simulink model "W09_E_weather"  (R2024b)
settings: Solver=ode4  StartTime=0  StopTime=T_final  FixedStep=h  RelTol=1e-3
values from neighbouring files (symbols this model uses):
  beta_c = pi/2    (= 1.57079632679)    [W09_0_setup.m]
  Delta = 5    [W09_0_setup.m]
  e_min = 0.3    [W09_0_setup.m]
  h = 0.02    [W09_0_setup.m]    (also in W09_1_build_vessel.m = add_line(sys, [a; via; b]); W09_metrics.m = V.h)
  hand_over = 1    [W09_0_setup.m]
  k_neg = cfg.k_neg    [W09_0_setup.m]
  k_pos = cfg.k_pos    [W09_0_setup.m]
  kappa = 0.3    [W09_0_setup.m]
  Kd = 100    [W09_0_setup.m]
  Kd_x = 60    [W09_0_setup.m]
  Ki_u = 200    [W09_0_setup.m]
  Ki_x = 3    [W09_0_setup.m]
  Kp = 300    [W09_0_setup.m]
  Kp_u = 200    [W09_0_setup.m]
  Kp_x = 30    [W09_0_setup.m]
  mp = 25    [W09_0_setup.m]
  N_max = min(2*cfg.y_pont*(cfg.k_pos*cfg.n_max^2 - X_max/2),              2*cfg.y_pont*(X_max/2 + cfg.k_neg*cfg.n_min^2))    [W09_0_setup.m]
  N_open = 2*cfg.y_pont*cfg.k_pos*cfg.n_max^2    [W09_0_setup.m]
  phi_i = mod(phi_i + phase_shift, 2*pi)    [W09_0_setup.m]
  R_arrive = 3    [W09_0_setup.m]
  rp = [0.05 0 -0.35]'    [W09_0_setup.m]
  T_hold = 30    [W09_0_setup.m]
  T_max = cfg.k_pos*cfg.n_max^2    [W09_0_setup.m]
  T_min = -cfg.k_neg*cfg.n_min^2    [W09_0_setup.m]
  u_d = 1.0    (= 1)    [W09_0_setup.m]
  use_ilos = 1    [W09_0_setup.m]
  use_Kd = 1    [W09_0_setup.m]
  use_Ki_u = 1    [W09_0_setup.m]
  use_pass = 1    [W09_0_setup.m]
  use_scale = 1    [W09_0_setup.m]
  use_ssa = 1    [W09_0_setup.m]
  use_vane = 1    [W09_0_setup.m]
  V_c = 0.3    [W09_0_setup.m]
  w0 = 2*pi/T0    (= 3.14159265359)    [W09_0_setup.m]
  wave_on = 1    [W09_0_setup.m]
  WP_E = [ 0 60 60]'    [W09_0_setup.m]
  WP_N = [60 60  0]'    [W09_0_setup.m]
  x0 = zeros(12,1)    [W09_0_setup.m]
  X_max = 120    [W09_0_setup.m]
  y_pont = cfg.y_pont    [W09_0_setup.m]
  zeta_d = 0.3    [W09_0_setup.m]
  zeta_n = 0.05    [W09_0_setup.m]
undefined symbols (not defined in the file or in its folder): a_i, k_w, w_i
settings Model: Creator=admin  LastModifiedBy=admin
settings DataIOCC: ReturnWorkspaceOutputs=off

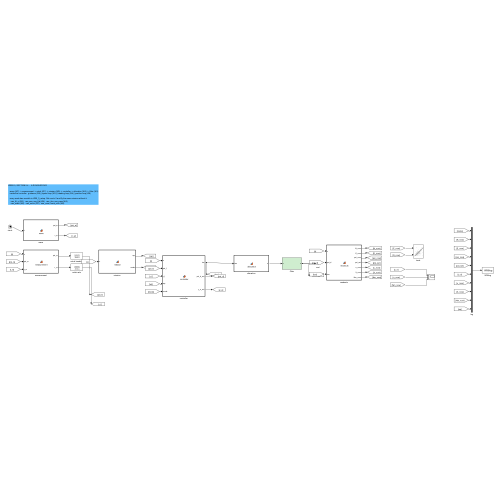
[thumbnail: Simulink's stored preview of the top-level diagram]
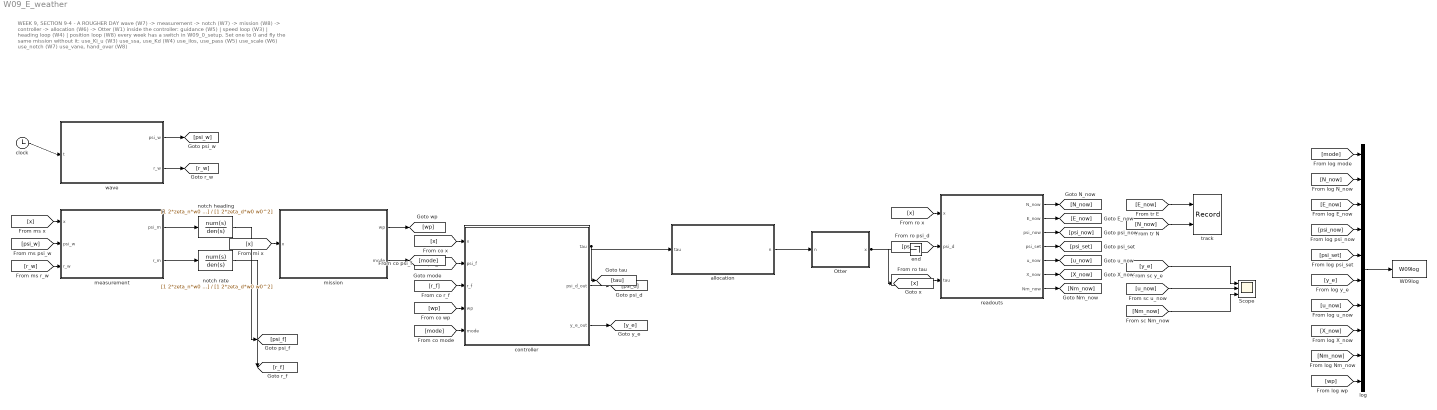
== system W09_E_weather ==
  note: WEEK 9, SECTION 9-4  -  A ROUGHER DAY
      |
      |    wave (W7) -> measurement -> notch (W7) -> mission (W8) -> controller -> allocation (W6) -> Otter (W1)
      |    inside the controller:  guidance (W5) | speed loop (W3) | heading loop (W4) | position loop (W8)
      |
      |    every week has a switch in W09_0_setup. Set one to 0 and fly the same mission without it:
      |      use_Ki_u (W3)   use_ssa, use_Kd (W4)   use_ilos, use_pass (W5)
      |      use_scale (W6)   use_notch (W7)   use_vane, hand_over (W8)
  Otter : Subsystem
  Scope : Scope  NumInputPorts=3
  W09log : ToWorkspace  VariableName=W09log  SaveFormat=Structure With Time  SampleTime=-1
  allocation : MATLAB Function  TreatAsAtomicUnit=on
  clock : Clock
  controller : MATLAB Function  TreatAsAtomicUnit=on
  end : Terminator
  log : Mux  Inputs=10
  measurement : MATLAB Function  TreatAsAtomicUnit=on
  mission : MATLAB Function  TreatAsAtomicUnit=on
  notch heading : TransferFcn  Numerator=[1 2*zeta_n*w0 w0^2]  Denominator=[1 2*zeta_d*w0 w0^2]
  notch rate : TransferFcn  Numerator=[1 2*zeta_n*w0 w0^2]  Denominator=[1 2*zeta_d*w0 w0^2]
  readouts : MATLAB Function  TreatAsAtomicUnit=on
  track : Record  FileSettingsInternal="{\"entries\":[{\"content\":{\"excelSettings\":{\"content\":{},\"type\":\"Streamout.ExcelSettings\"}},\"type\":\"Streamout.FileSettingStorage\",\"uuid\":\"\"}],\"packageUris\":[\"http:\\/\\/schema.mathworks.com\\/mf0\\/streamout_blocks\\/R2020a\"],\"version\":\"1.0\"}"  Layout=[1 1]  SignalsInternal="{\"entries\":[{\"content\":{\"signals\":[{\"content\":{\"blockPath\":[],\"dimensions\":[1],\"domain\":\"\",\"lineColor\":\"#a2142f\",\"plots\":[ 1 ],\"port\":1,\"signalID\":1,\"signalName\":\"XY Graph:1\"},\"type\":\"RecordBlkView.Signal\",\"uuid\":\"\"},{\"content\":{\"blockPath\":[],\"dimensions\":[1],\"domain\":\"\",\"lineColor\":\"#139fff\",\"plots\":[ 1 ],\"port\":2,\"signalID\":2,\"signalName\":\"XY Graph:2\"},\"type\":\"RecordBlkView.Signal\",\"uuid\":\"\"}]},\"type\":\"RecordBlkView.InputSignals\",\"uuid\":\"\"}],\"packageUris\":[\"http:\\/\\/schema.mathworks.com\\/mf0\\/streamout_blocks\\/R2020a\"],\"version\":\"1.0\"}"  VisualizationBindings="{\"xyplotplugin\":{\"info\":[{\"series\":[{\"bindingParametersList\":[{\"parameter\":\"X-Axis\",\"signalID\":1,\"signalName\":\"XY Graph:1\"},{\"parameter\":\"Y-Axis\",\"signalID\":2,\"signalName\":\"XY Graph:2\"}],\"seriesID\":0}],\"subplotID\":1}]}}"  CompatibilityTag=XY
  wave : MATLAB Function  TreatAsAtomicUnit=on
  wires:
  clock/1 -> wave/1(t)
  wave/1(psi_w) -> [psi_w]
  wave/2(r_w) -> [r_w]
  [x] -> measurement/1(x)
  [psi_w] -> measurement/2(psi_w)
  [r_w] -> measurement/3(r_w)
  measurement/1(psi_m) -> notch heading/1
  notch heading/1 -> [psi_f]
  measurement/2(r_m) -> notch rate/1
  notch rate/1 -> [r_f]
  [x] -> mission/1(x)
  mission/1(wp) -> [wp]
  mission/2(mode) -> [mode]
  [x] -> controller/1(x)
  [psi_f] -> controller/2(psi_f)
  [r_f] -> controller/3(r_f)
  [wp] -> controller/4(wp)
  [mode] -> controller/5(mode)
  controller/1(tau) -> [tau], allocation/1(tau)
  controller/2(psi_d_out) -> [psi_d]
  controller/3(y_e_out) -> [y_e]
  allocation/1(n) -> Otter/1(n)
  Otter/1(x) -> [x], end/1
  [x] -> readouts/1(x)
  [psi_d] -> readouts/2(psi_d)
  [tau] -> readouts/3(tau)
  readouts/1(N_now) -> [N_now]
  readouts/2(E_now) -> [E_now]
  readouts/3(psi_now) -> [psi_now]
  readouts/4(psi_set) -> [psi_set]
  readouts/5(u_now) -> [u_now]
  readouts/6(X_now) -> [X_now]
  readouts/7(Nm_now) -> [Nm_now]
  [E_now] -> track/1
  [N_now] -> track/2
  [y_e] -> Scope/1
  [u_now] -> Scope/2
  [Nm_now] -> Scope/3
  [mode] -> log/1
  [N_now] -> log/2
  [E_now] -> log/3
  [psi_now] -> log/4
  [psi_set] -> log/5
  [y_e] -> log/6
  [u_now] -> log/7
  [X_now] -> log/8
  [Nm_now] -> log/9
  [wp] -> log/10
  log/1 -> W09log/1

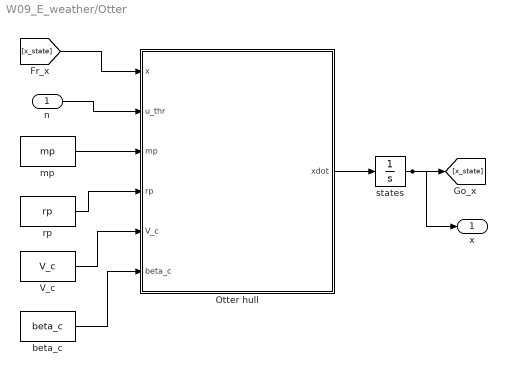
== system W09_E_weather/Otter ==
  n : Inport
  Otter hull : MATLAB Function  TreatAsAtomicUnit=on
  V_c : Constant  Value=V_c
  beta_c : Constant  Value=beta_c
  mp : Constant  Value=mp
  rp : Constant  Value=rp
  states : Integrator  InitialCondition=x0
  x : Outport
  wires:
  states/1 -> [x_state], x/1
  Otter hull/1(xdot) -> states/1
  [x_state] -> Otter hull/1(x)
  n/1 -> Otter hull/2(u_thr)
  mp/1 -> Otter hull/3(mp)
  rp/1 -> Otter hull/4(rp)
  V_c/1 -> Otter hull/5(V_c)
  beta_c/1 -> Otter hull/6(beta_c)

== matlab function W09_E_weather/allocation ==
  data: tau input; n output double size=[2 1]; y_pont parameter; k_pos parameter; k_neg parameter; T_max parameter; T_min parameter; use_scale parameter
function n = allocation(tau, y_pont, k_pos, k_neg, T_max, T_min, use_scale)
%#codegen
%  6주차의 배분. use_scale = 0 이면 §6-6 의 자르기로 돌아간다.
T1 = tau(1)/2 + tau(2)/(2*y_pont);
T2 = tau(1)/2 - tau(2)/(2*y_pont);
if use_scale ~= 0
    %  6주차 §6-6: 둘을 같은 비율로 줄이면 방향이 지켜진다 / scale, and the direction survives
    s = 1;
    if T1 > T_max, s = min(s, T_max/T1); end
    if T2 > T_max, s = min(s, T_max/T2); end
    if T1 < T_min, s = min(s, T_min/T1); end
    if T2 < T_min, s = min(s, T_min/T2); end
    T1 = s*T1;  T2 = s*T2;
else
    %  각각 따로 자른다. 한쪽만 잘리면 두 추진기의 차가 달라지고,
    %  그래서 **명령한 모멘트가 나오지 않는다** (6주차 §6-6).
    %  Clip each on its own: when only one is clipped the difference changes,
    %  so the moment that comes out is not the moment that was asked for.
    T1 = min(max(T1, T_min), T_max);
    T2 = min(max(T2, T_min), T_max);
end
k1 = k_pos;  if T1 < 0, k1 = k_neg; end
k2 = k_pos;  if T2 < 0, k2 = k_neg; end
n = [sign(T1)*sqrt(abs(T1)/k1); sign(T2)*sqrt(abs(T2)/k2)];

== matlab function W09_E_weather/Otter/Otter hull ==
  data: x input; xdot output double size=[12 1]; u_thr input; mp input; rp input; V_c input; beta_c input
function xdot = otter_hull(x, u_thr, mp, rp, V_c, beta_c)
% Fossen's otter.m, called unchanged from Tools/MSS/VESSELS.
%
%   x       12 states, fed back from the integrator
%   u_thr   propeller shaft speeds [rad/s]
%
% otter.m is not written for code generation, so the call is extrinsic and
% xdot has to be pre-sized for Simulink to know the output width.
coder.extrinsic('otter');

xdot = zeros(12,1);
xdot = otter(x, u_thr, mp, rp, V_c, beta_c);
end

== matlab function W09_E_weather/readouts ==
  data: x input; N_now output double size=[1 1]; psi_d input; tau input; E_now output; psi_now output; psi_set output; u_now output; X_now output; Nm_now output
function [N_now, E_now, psi_now, psi_set, u_now, X_now, Nm_now] = readouts(x, psi_d, tau)
%#codegen
N_now = x(7);  E_now = x(8);  psi_now = x(12)*180/pi;  psi_set = psi_d*180/pi;
u_now = x(1);  X_now = tau(1);  Nm_now = tau(2);

== matlab function W09_E_weather/measurement ==
  data: x input; psi_m output double size=[1 1]; psi_w input; r_w input; r_m output
function [psi_m, r_m] = measurement(x, psi_w, r_w)
%#codegen
%  제어기가 보는 것 = 배가 하는 것 + 1차 파랑 (7주차 §7-2)
psi_m = x(12)*180/pi + psi_w;
r_m   = x(6)*180/pi  + r_w;

== matlab function W09_E_weather/wave ==
  data: t input; psi_w output double size=[1 1]; r_w output; w_i parameter; a_i parameter; phi_i parameter; k_w parameter; wave_on parameter
function [psi_w, r_w] = wave(t, w_i, a_i, phi_i, k_w, wave_on)
%#codegen
%  7주차의 바다 그대로 / the sea of Week 7, unchanged
psi_w = 0;  r_w = 0;
if wave_on ~= 0
    for i = 1:numel(w_i)
        psi_w = psi_w + k_w*a_i(i)*sin(w_i(i)*t + phi_i(i));
        r_w   = r_w   + k_w*a_i(i)*w_i(i)*cos(w_i(i)*t + phi_i(i));
    end
end

== matlab function W09_E_weather/mission ==
  settings: updateMethod=DISCRETE  sampleTime=h
  data: x input; wp output double size=[1 1]; mode output; WP_N parameter; WP_E parameter; R_arrive parameter; T_hold parameter; use_pass parameter; h parameter
function [wp, mode] = mission(x, WP_N, WP_E, R_arrive, T_hold, use_pass, h)
%#codegen
%  8주차 §8-5 의 상태기계. 규칙은 둘뿐이다.
%  The state machine of Week 8 §8-5: two rules only.
persistent k mode_ held
if isempty(k), k = 1; mode_ = 1; held = 0; end
d = hypot(WP_N(k) - x(7), WP_E(k) - x(8));
%  도착 판정 / the arrival test
%    원 안에 들어왔는가 — 빠르게 지나가면 놓칠 수 있다 (§9-5)
%    그리고 5주차의 판정: 다리 방향으로 남은 거리가 음수가 되었는가, 즉 지나갔는가
%    the acceptance circle, which a fast pass can miss, and the along-track test
%    of Week 5: the distance still to run along the leg has gone negative
if k > 1, N0 = WP_N(k-1);  E0 = WP_E(k-1);  else, N0 = 0;  E0 = 0;  end
pi_p   = atan2(WP_E(k) - E0, WP_N(k) - N0);
x_left = (WP_N(k) - x(7))*cos(pi_p) + (WP_E(k) - x(8))*sin(pi_p);
reached = d < R_arrive || (use_pass ~= 0 && x_left < 0);
if mode_ == 1 && reached
    mode_ = 2;  held = 0;
elseif mode_ == 2
    held = held + h;
    if held >= T_hold
        if k < numel(WP_N), k = k + 1;  mode_ = 1;  else, mode_ = 3; end
    end
end
wp = k;  mode = mode_;

== matlab function W09_E_weather/controller ==
  settings: updateMethod=DISCRETE  sampleTime=h
  data: x input; tau output double size=[2 1]; psi_f input; r_f input; wp input; mode input; psi_d_out output; y_e_out output; WP_N parameter; WP_E parameter; Delta parameter; kappa parameter; u_d parameter; Kp_u parameter; Ki_u parameter; Kp parameter; Kd parameter; Kp_x parameter; Ki_x parameter; Kd_x parameter; e_min parameter; X_max parameter; N_max parameter; N_open parameter; use_Ki_u parameter; use_ssa parameter; use_Kd parameter; use_ilos parameter; use_scale parameter; use_vane parameter; hand_over parameter; h parameter
function [tau, psi_d_out, y_e_out] = controller(x, psi_f, r_f, wp, mode, WP_N, WP_E, Delta, kappa, u_d, Kp_u, Ki_u, Kp, Kd, Kp_x, Ki_x, Kd_x, e_min, X_max, N_max, N_open, use_Ki_u, use_ssa, use_Kd, use_ilos, use_scale, use_vane, hand_over, h)
%#codegen
%  여덟 주차가 한 블록에 들어 있다. 모드에 따라 어느 줄이 도는지가 달라질 뿐이다.
%  Eight weeks in one block; the mode decides which lines run.
psi = x(12);  u = x(1);  v = x(2);
psi_m = psi_f*pi/180;  r_m = r_f*pi/180;      % 노치를 지난 계측 (7주차)
k = wp;  y_e = 0;
persistent I_u y_int In Ie psi_last
if isempty(I_u), I_u = 0; y_int = 0; In = 0; Ie = 0; psi_last = psi; end
if mode == 1
    %  ── 이동 / transit ────────────────────────────────────────────────
    %  5주차: 앞 지점에서 이 지점으로 가는 다리 위의 횡방향 오차와 LOS/ILOS
    %  Week 5: the cross-track error of the active leg, and the LOS or ILOS law
    if k > 1, N0 = WP_N(k-1);  E0 = WP_E(k-1);  else, N0 = 0;  E0 = 0;  end
    pi_p = atan2(WP_E(k) - E0, WP_N(k) - N0);
    y_e  = -(x(7) - N0)*sin(pi_p) + (x(8) - E0)*cos(pi_p);
    if use_ilos ~= 0
        psi_d = pi_p - atan((y_e + kappa*y_int)/Delta);
        y_int = y_int + h*Delta*y_e/(Delta^2 + (y_e + kappa*y_int)^2);
    else
        psi_d = pi_p - atan(y_e/Delta);
    end
    %  3주차: 속도 루프 / Week 3: the speed loop
    eu = u_d - u;
    X  = Kp_u*eu + I_u;
    X  = min(max(X, -X_max), X_max);
    if use_Ki_u ~= 0 && abs(X) < X_max - 1e-9, I_u = I_u + h*Ki_u*eu; end
    if hand_over ~= 0, In = 0;  Ie = 0; end   % 8주차: 유지를 깨끗하게 시작하도록
    psi_last = psi_d;                         % 유지가 이어받는 선수각 / the heading a hold inherits
else
    %  ── 유지 / hold ──────────────────────────────────────────────────
    %  8주차: 위치 PID 를 NED 에서 풀고, 그 힘의 방향으로 뱃머리를 둔다
    e_n = WP_N(k) - x(7);  e_e = WP_E(k) - x(8);
    v_n = u*cos(psi) - v*sin(psi);  v_e = u*sin(psi) + v*cos(psi);
    f_n = Kp_x*e_n + In - Kd_x*v_n;
    f_e = Kp_x*e_e + Ie - Kd_x*v_e;
    if use_vane ~= 0
        if hypot(f_n, f_e) > e_min, psi_last = atan2(f_e, f_n); end
        psi_d = psi_last;
    else
        psi_d = psi_last;                      % 도착했을 때의 선수각을 그대로
    end
    X = f_n*cos(psi) + f_e*sin(psi);
    X = min(max(X, -X_max), X_max);
    if abs(X) < X_max - 1e-9
        In = In + h*Ki_x*e_n;  Ie = Ie + h*Ki_x*e_e;
    end
    I_u = 0;
end
%  ── 4주차: 선수각 / Week 4: the heading loop ─────────────────────────
%  4주차 §4-6 의 ssa. 끄면 이음매에서 오차가 한 바퀴만큼 뛴다.
%  The ssa of Week 4 §4-6. Switched off, the error jumps by a whole turn at the seam.
if use_ssa ~= 0
    ee = atan2(sin(psi_d - psi_m), cos(psi_d - psi_m));
else
    ee = psi_d - psi_m;
end
N  = Kp*ee;
if use_Kd ~= 0, N = N - Kd*r_m; end
%  6주차: 요 한계는 **이미 쓰고 있는 전진력에 달려 있다**. use_scale = 0 은 그 결합을
%  잊은 설계다 — 전진력이 0 일 때의 한계 N_open 을 그대로 쓴다.
%  Week 6: the yaw limit depends on the surge already spent. use_scale = 0 is the
%  design that forgets the coupling and keeps N_open, the limit at zero surge.
N_lim = N_max;
if use_scale == 0, N_lim = N_open; end
N  = min(max(N, -N_lim), N_lim);
if mode == 3, X = 0;  N = 0; end
tau = [X; N];  psi_d_out = psi_d;  y_e_out = y_e;
